simulink model "Bixler"  (R2019b)
settings: Solver=ode45  StartTime=0.0  StopTime=60  RelTol=1e-6  AbsTol=1e-8
PostLoadFcn:
  | parameters_main
  | write_init_cond
StartFcn:
  | write_init_cond
  | disp('Simulating...');
StopFcn:
  | timetime = datestr(datetime('now','Format','hh:mm'));
  | disp(['End of Simulation.       ', timetime]);
  | clear timetime
undefined symbols (not defined in the file): Aero, APlane, Bxl, C, Ctr, deg, DiscIntNeverNeededParam, Earth, F, Guid, Init, Light, MIL, Path, rad, s, Trim, Utility, WGS84
libraries: aerolibconvert2 x39, simulink x14, dspsigops x6, simulink_extras x3, aerolibtransform2 x2, aerolibasang x2, aerolibfltsims x2, shared6dof x1, aerolibadyn x1, aerolibwind2 x1, aerolibanim x1, realtime_pacer_lib x1
(part 4 of 5)

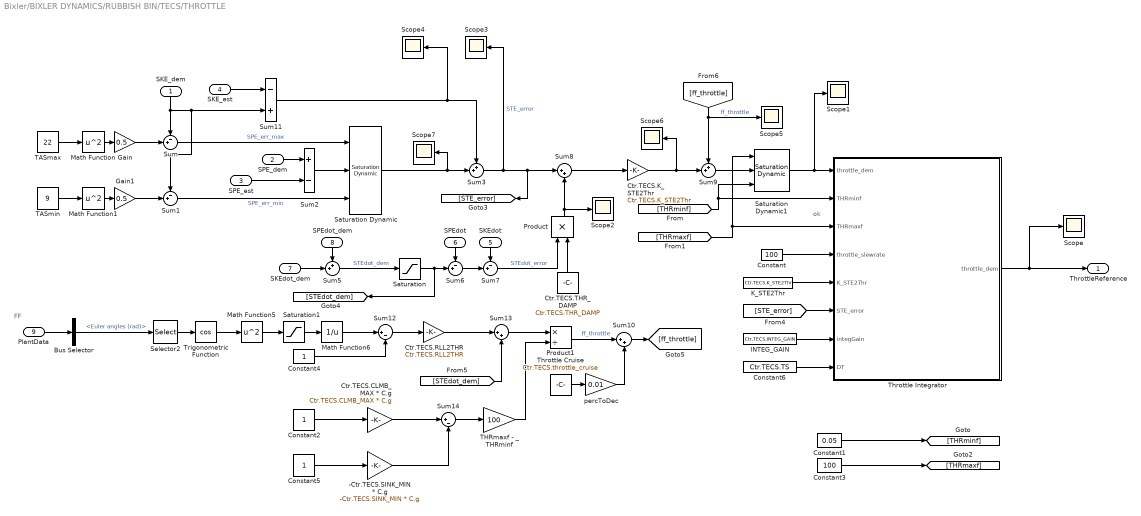
== system Bixler/BIXLER DYNAMICS/RUBBISH BIN/TECS/THROTTLE ==
  note: FF
  note: ok
  SKE_dem : Inport
  SPE_dem : Inport  Port=2
  SPE_est : Inport  Port=3
  SKE_est : Inport  Port=4
  SKEdot : Inport  Port=5
  SPEdot : Inport  Port=6
  SKEdot_dem : Inport  Port=7
  SPEdot_dem : Inport  Port=8
  PlantData : Inport  Port=9
  -Ctr.TECS.SINK_MIN * C.g : Gain  Gain=-Ctr.TECS.SINK_MIN * C.g
  Bus Selector : BusSelector  OutputSignals=Euler angles (rad)
  Constant : Constant  Value=100
  Constant1 : Constant  Value=0.05
  Constant2 : Constant
  Constant3 : Constant  Value=100
  Constant4 : Constant
  Constant5 : Constant
  Constant6 : Constant  Value=Ctr.TECS.TS
  Ctr.TECS.CLMB_MAX * C.g : Gain  Gain=Ctr.TECS.CLMB_MAX * C.g
  Ctr.TECS.K_STE2Thr : Gain  Gain=Ctr.TECS.K_STE2Thr
  Ctr.TECS.RLL2THR : Gain  Gain=Ctr.TECS.RLL2THR
  Ctr.TECS.THR_DAMP : Constant  Value=Ctr.TECS.THR_DAMP
  Gain : Gain  Gain=0.5
  Gain1 : Gain  Gain=0.5
  INTEG_GAIN : Constant  Value=Ctr.TECS.INTEG_GAIN
  K_STE2Thr : Constant  Value=Ctr.TECS.K_STE2Thr
  Math Function : Math  Operator=square  SignedPower=on  SaturateOnIntegerOverflow=on
  Math Function1 : Math  Operator=square  SignedPower=on  SaturateOnIntegerOverflow=on
  Math Function5 : Math  Operator=square  SignedPower=on  SaturateOnIntegerOverflow=on
  Math Function6 : Math  Operator=reciprocal  SignedPower=on  SaturateOnIntegerOverflow=on
  Product : Product
  Product1 : Product  Inputs=*/
  Saturation : Saturate  UpperLimit=Ctr.TECS.STEdot_max  LowerLimit=Ctr.TECS.STEdot_min
  Saturation Dynamic : simulink/Discontinuities/Saturation Dynamic  OutMin=[]  OutMax=[]  OutDataTypeStr=Inherit: Same as second input  OutDataType=fixdt(1, 16)  OutScaling=2^-10  DoSatur=off
  Saturation Dynamic1 : simulink/Discontinuities/Saturation Dynamic  OutMin=[]  OutMax=[]  OutDataTypeStr=Inherit: Same as second input  OutDataType=fixdt(1, 16)  OutScaling=2^-10  DoSatur=off
  Saturation1 : Saturate  UpperLimit=1  LowerLimit=0.1
  Scope{,1..7} (8 alike) : Scope
  Selector2 : Selector  InputPortWidth=3  IndexOptions=Index vector (dialog)  Indices=1  OutputSizes=1
  Sum{,1,6..7} (4 alike) : Sum  Inputs=-+|
  Sum10 : Sum  Inputs=|++
  Sum11 : Sum  Inputs=-+
  Sum12 : Sum  Inputs=|+-
  Sum13 : Sum  Inputs=|++
  Sum14 : Sum  Inputs=|+-
  Sum2 : Sum  Inputs=+-
  Sum3 : Sum  Inputs=++|
  Sum5 : Sum  Inputs=++|
  Sum8 : Sum  Inputs=|++
  Sum9 : Sum  Inputs=++|
  TASmax : Constant  Value=22
  TASmin : Constant  Value=9
  THRmaxf - _THRminf : Gain  Gain=100
  Throttle Cruise : Constant  Value=Ctr.TECS.throttle_cruise
  Throttle Integrator : MATLAB Function  TreatAsAtomicUnit=on
  Trigonometric Function : Trigonometry  Operator=cos
  percToDec : Gain  Gain=0.01
  ThrottleReference : Outport  VectorParamsAs1DForOutWhenUnconnected=off
  wires:
  Throttle Integrator/1(throttle_dem) -> Scope/1, ThrottleReference/1
  Constant6/1 -> Throttle Integrator/8(DT)
  SKE_dem/1 -> Sum11/2, Sum1/1, Sum/1
  Math Function1/1 -> Gain1/1
  TASmin/1 -> Math Function1/1
  Sum1/1 -> Saturation Dynamic/3  "SPE_err_min"
  Gain1/1 -> Sum1/2
  TASmax/1 -> Math Function/1
  Sum5/1 -> Saturation/1  "STEdot_dem"
  SPEdot/1 -> Sum6/1
  Saturation Dynamic1/1 -> Scope1/1, Throttle Integrator/1("throttle_dem ")
  Product/1 -> Sum8/2, Scope2/1
  Saturation/1 -> [STEdot_dem], Sum6/2
  Ctr.TECS.THR_DAMP/1 -> Product/2
  SPE_est/1 -> Sum2/2
  Sum6/1 -> Sum7/2
  Sum3/1 -> Scope3/1, [STE_error], Sum8/1  "STE_error"
  SPEdot_dem/1 -> Sum5/1
  SKEdot_dem/1 -> Sum5/2
  SKE_est/1 -> Sum11/1
  Sum7/1 -> Product/1  "STEdot_error"
  Sum2/1 -> Saturation Dynamic/2
  SKEdot/1 -> Sum7/1
  Sum9/1 -> Saturation Dynamic1/2
  Sum/1 -> Saturation Dynamic/1  "SPE_err_max"
  Gain/1 -> Sum/2
  Math Function/1 -> Gain/1
  Constant1/1 -> [THRminf]
  Constant3/1 -> [THRmaxf]
  [THRminf] -> Throttle Integrator/2(THRminf), Saturation Dynamic1/3
  [THRmaxf] -> Saturation Dynamic1/1, Throttle Integrator/3(THRmaxf)
  Constant/1 -> Throttle Integrator/4(throttle_slewrate)
  [STE_error] -> Throttle Integrator/6(STE_error)
  INTEG_GAIN/1 -> Throttle Integrator/7(integGain)
  SPE_dem/1 -> Sum2/1
  PlantData/1 -> Bus Selector/1
  Bus Selector/1 -> Selector2/1  "<Euler angles (rad)>"
  Selector2/1 -> Trigonometric Function/1
  Saturation1/1 -> Math Function6/1
  Math Function6/1 -> Sum12/1
  Constant4/1 -> Sum12/2
  Sum12/1 -> Ctr.TECS.RLL2THR/1
  Ctr.TECS.RLL2THR/1 -> Sum13/1
  [STEdot_dem] -> Sum13/2
  Ctr.TECS.K_STE2Thr/1 -> Scope6/1, Sum9/2
  K_STE2Thr/1 -> Throttle Integrator/5(K_STE2Thr)
  [ff_throttle] -> Sum9/1, Scope5/1  "ff_throttle"
  Sum8/1 -> Ctr.TECS.K_STE2Thr/1
  Math Function5/1 -> Saturation1/1
  Sum13/1 -> Product1/1
  Throttle Cruise/1 -> percToDec/1
  Constant2/1 -> Ctr.TECS.CLMB_MAX * C.g/1
  Constant5/1 -> -Ctr.TECS.SINK_MIN * C.g/1
  Ctr.TECS.CLMB_MAX * C.g/1 -> Sum14/1
  -Ctr.TECS.SINK_MIN * C.g/1 -> Sum14/2
  Sum14/1 -> THRmaxf - _THRminf/1
  THRmaxf - _THRminf/1 -> Product1/2
  Product1/1 -> Sum10/1  "ff_throttle"
  Sum10/1 -> [ff_throttle]
  Sum11/1 -> Scope4/1, Sum3/1
  Saturation Dynamic/1 -> Scope7/1, Sum3/2
  percToDec/1 -> Sum10/2
  Trigonometric Function/1 -> Math Function5/1

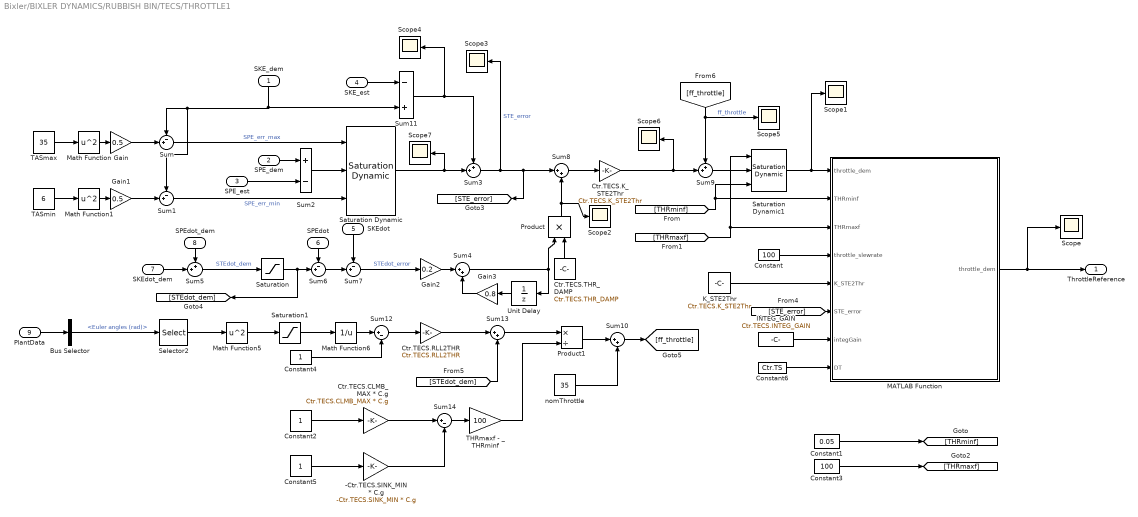
== system Bixler/BIXLER DYNAMICS/RUBBISH BIN/TECS/THROTTLE1 ==
  SKE_dem : Inport
  SPE_dem : Inport  Port=2
  SPE_est : Inport  Port=3
  SKE_est : Inport  Port=4
  SKEdot : Inport  Port=5
  SPEdot : Inport  Port=6
  SKEdot_dem : Inport  Port=7
  SPEdot_dem : Inport  Port=8
  PlantData : Inport  Port=9
  -Ctr.TECS.SINK_MIN * C.g : Gain  Gain=-Ctr.TECS.SINK_MIN * C.g
  Bus Selector : BusSelector  OutputSignals=Euler angles (rad)
  Constant : Constant  Value=100
  Constant1 : Constant  Value=0.05
  Constant2 : Constant
  Constant3 : Constant  Value=100
  Constant4 : Constant
  Constant5 : Constant
  Constant6 : Constant  Value=Ctr.TS
  Ctr.TECS.CLMB_MAX * C.g : Gain  Gain=Ctr.TECS.CLMB_MAX * C.g
  Ctr.TECS.K_STE2Thr : Gain  Gain=Ctr.TECS.K_STE2Thr
  Ctr.TECS.RLL2THR : Gain  Gain=Ctr.TECS.RLL2THR
  Ctr.TECS.THR_DAMP : Constant  Value=Ctr.TECS.THR_DAMP
  Gain : Gain  Gain=0.5
  Gain1 : Gain  Gain=0.5
  Gain2 : Gain  Gain=0.2
  Gain3 : Gain  Gain=0.8
  INTEG_GAIN : Constant  Value=Ctr.TECS.INTEG_GAIN
  K_STE2Thr : Constant  Value=Ctr.TECS.K_STE2Thr
  MATLAB Function : MATLAB Function  TreatAsAtomicUnit=on
  Math Function : Math  Operator=square  SignedPower=on  SaturateOnIntegerOverflow=on
  Math Function1 : Math  Operator=square  SignedPower=on  SaturateOnIntegerOverflow=on
  Math Function5 : Math  Operator=square  SignedPower=on  SaturateOnIntegerOverflow=on
  Math Function6 : Math  Operator=reciprocal  SignedPower=on  SaturateOnIntegerOverflow=on
  Product : Product
  Product1 : Product  Inputs=*/
  Saturation : Saturate  UpperLimit=Ctr.TECS.STEdot_max  LowerLimit=Ctr.TECS.STEdot_min
  Saturation Dynamic : simulink/Discontinuities/Saturation Dynamic  OutMin=[]  OutMax=[]  OutDataTypeStr=Inherit: Same as second input  OutDataType=fixdt(1, 16)  OutScaling=2^-10  DoSatur=off
  Saturation Dynamic1 : simulink/Discontinuities/Saturation Dynamic  OutMin=[]  OutMax=[]  OutDataTypeStr=Inherit: Same as second input  OutDataType=fixdt(1, 16)  OutScaling=2^-10  DoSatur=off
  Saturation1 : Saturate  UpperLimit=1  LowerLimit=0.1
  Scope{,1..7} (8 alike) : Scope
  Selector2 : Selector  InputPortWidth=3  IndexOptions=Index vector (dialog)  Indices=1  OutputSizes=1
  Sum{,1,6..7} (4 alike) : Sum  Inputs=-+|
  Sum{4,8,10,13} (4 alike) : Sum  Inputs=|++
  Sum11 : Sum  Inputs=-+
  Sum12 : Sum  Inputs=|+-
  Sum14 : Sum  Inputs=|+-
  Sum2 : Sum  Inputs=+-
  Sum3 : Sum  Inputs=++|
  Sum5 : Sum  Inputs=++|
  Sum9 : Sum  Inputs=++|
  TASmax : Constant  Value=35
  TASmin : Constant  Value=6
  THRmaxf - _THRminf : Gain  Gain=100
  Unit Delay : UnitDelay  SampleTime=Ctr.TS  HasFrameUpgradeWarning=on
  nomThrottle : Constant  Value=35
  ThrottleReference : Outport  VectorParamsAs1DForOutWhenUnconnected=off
  wires:
  MATLAB Function/1(throttle_dem) -> Scope/1, ThrottleReference/1
  Constant6/1 -> MATLAB Function/8(DT)
  SKE_dem/1 -> Sum/1, Sum1/1, Sum11/2
  Math Function1/1 -> Gain1/1
  TASmin/1 -> Math Function1/1
  Sum1/1 -> Saturation Dynamic/3  "SPE_err_min"
  Gain1/1 -> Sum1/2
  TASmax/1 -> Math Function/1
  Sum5/1 -> Saturation/1  "STEdot_dem"
  SPEdot/1 -> Sum6/1
  Saturation Dynamic1/1 -> Scope1/1, MATLAB Function/1("throttle_dem ")
  Product/1 -> Scope2/1, Sum8/2
  Saturation/1 -> [STEdot_dem], Sum6/2
  Ctr.TECS.THR_DAMP/1 -> Product/2
  SPE_est/1 -> Sum2/2
  Sum6/1 -> Sum7/2
  Sum3/1 -> Scope3/1, [STE_error], Sum8/1  "STE_error"
  SPEdot_dem/1 -> Sum5/1
  SKEdot_dem/1 -> Sum5/2
  SKE_est/1 -> Sum11/1
  Sum7/1 -> Gain2/1  "STEdot_error"
  Sum2/1 -> Saturation Dynamic/2
  SKEdot/1 -> Sum7/1
  Sum9/1 -> Saturation Dynamic1/2
  Sum/1 -> Saturation Dynamic/1  "SPE_err_max"
  Gain/1 -> Sum/2
  Math Function/1 -> Gain/1
  Constant1/1 -> [THRminf]
  Constant3/1 -> [THRmaxf]
  [THRminf] -> MATLAB Function/2(THRminf), Saturation Dynamic1/3
  [THRmaxf] -> Saturation Dynamic1/1, MATLAB Function/3(THRmaxf)
  Constant/1 -> MATLAB Function/4(throttle_slewrate)
  [STE_error] -> MATLAB Function/6(STE_error)
  INTEG_GAIN/1 -> MATLAB Function/7(integGain)
  SPE_dem/1 -> Sum2/1
  PlantData/1 -> Bus Selector/1
  Bus Selector/1 -> Selector2/1  "<Euler angles (rad)>"
  Selector2/1 -> Math Function5/1
  Saturation1/1 -> Math Function6/1
  Math Function6/1 -> Sum12/1
  Constant4/1 -> Sum12/2
  Sum12/1 -> Ctr.TECS.RLL2THR/1
  Ctr.TECS.RLL2THR/1 -> Sum13/1
  [STEdot_dem] -> Sum13/2
  Ctr.TECS.K_STE2Thr/1 -> Scope6/1, Sum9/2
  K_STE2Thr/1 -> MATLAB Function/5(K_STE2Thr)
  [ff_throttle] -> Sum9/1, Scope5/1  "ff_throttle"
  Sum8/1 -> Ctr.TECS.K_STE2Thr/1
  Math Function5/1 -> Saturation1/1
  Sum13/1 -> Product1/1
  nomThrottle/1 -> Sum10/2
  Constant2/1 -> Ctr.TECS.CLMB_MAX * C.g/1
  Constant5/1 -> -Ctr.TECS.SINK_MIN * C.g/1
  Ctr.TECS.CLMB_MAX * C.g/1 -> Sum14/1
  -Ctr.TECS.SINK_MIN * C.g/1 -> Sum14/2
  Sum14/1 -> THRmaxf - _THRminf/1
  THRmaxf - _THRminf/1 -> Product1/2
  Product1/1 -> Sum10/1
  Sum10/1 -> [ff_throttle]
  Sum11/1 -> Scope4/1, Sum3/1
  Gain2/1 -> Sum4/1
  Gain3/1 -> Sum4/2
  Unit Delay/1 -> Gain3/1
  Sum4/1 -> Unit Delay/1, Product/1
  Saturation Dynamic/1 -> Scope7/1, Sum3/2

== system Bixler/BIXLER DYNAMICS/Vehicle Airframe/Aerodynamics/Aerodynamic Coefficients ==
  PlantData : Inport
  Va : Inport  Port=2
  alpha(rad) : Inport  Port=3
  beta(rad) : Inport  Port=4
  Alpha Prelookup : PreLookup  BreakpointsData=Aero.alpha_vector  BeginIndexSearchUsingPreviousIndexResult=on  ExtrapMethod=Linear  RemoveProtectionInput=on
  Angle Conversion : aerolibconvert2/Angle Conversion  IU=rad  OU=deg
  Bus Selector : BusSelector  OutputSignals=Angular rates (body) (rad/s)
  Demux1 : Demux  Outputs=3
  Forces : Subsystem
  Goto Tag Visibility : GotoTagVisibility  GotoTag=pRad
  Goto Tag Visibility1 : GotoTagVisibility  GotoTag=qRad
  Goto Tag Visibility2 : GotoTagVisibility  GotoTag=rRad
  Goto Tag Visibility3 : GotoTagVisibility  GotoTag=BetaRad
  Moments : Subsystem
  Mux : Mux  Inputs=6
  Coeff : Outport  VectorParamsAs1DForOutWhenUnconnected=off
  tag scope: BetaRad=scoped, Va=global, alphaRad=scoped, pRad=scoped, qRad=scoped, rRad=scoped
  wires:
  Alpha Prelookup/2 -> Moments/2(alpha_f), Forces/2(alpha_f)  "f"
  alpha(rad)/1 -> [alphaRad], Angle Conversion/1
  PlantData/1 -> Bus Selector/1
  Forces/1(CD) -> Mux/1
  Forces/2(Cy) -> Mux/2
  Moments/1(Cl) -> Mux/4
  Demux1/3 -> [rRad]  "yaw_rate"
  Angle Conversion/1 -> Alpha Prelookup/1
  Demux1/2 -> [qRad]  "pitch_rate"
  beta(rad)/1 -> [BetaRad]
  Alpha Prelookup/1 -> Moments/1(alpha_k), Forces/1(alpha_k)  "k"
  Demux1/1 -> [pRad]  "roll_rate"
  Forces/3(CL) -> Mux/3
  Moments/3(Cn) -> Mux/6
  Moments/2(Cm) -> Mux/5
  Mux/1 -> Coeff/1
  Bus Selector/1 -> Demux1/1  "<Angular rates (body) (rad/s)>"
  Va/1 -> [Va]

== system Bixler/BIXLER DYNAMICS/Vehicle Airframe/Aerodynamics/ControlIncrements ==
  DerCond : Inport
  Control : Inport  Port=2
  Ailerons : Subsystem
  Alpha : PreLookup  BreakpointsData=Aero.alpha_vector  BeginIndexSearchUsingPreviousIndexResult=on  ExtrapMethod=Linear  RemoveProtectionInput=on
  Angle Conversion : aerolibconvert2/Angle Conversion  IU=rad  OU=deg
  Bus Selector : BusSelector  OutputSignals=alpha
  Bus Selector1 : BusSelector  OutputSignals=delta_ail,delta_elev,delta_rudd
  Elevator : Subsystem
  Rudder : Subsystem
  Cn_ail : Outport  VectorParamsAs1DForOutWhenUnconnected=off
  Cl_ail : Outport  Port=2  VectorParamsAs1DForOutWhenUnconnected=off
  CD_elev : Outport  Port=3  VectorParamsAs1DForOutWhenUnconnected=off
  CL_elev : Outport  Port=4  VectorParamsAs1DForOutWhenUnconnected=off
  Cm_elev : Outport  Port=5  VectorParamsAs1DForOutWhenUnconnected=off
  Cy_rudd : Outport  Port=6  VectorParamsAs1DForOutWhenUnconnected=off
  Cl_rudd : Outport  Port=7  VectorParamsAs1DForOutWhenUnconnected=off
  Cn_rudd : Outport  Port=8  VectorParamsAs1DForOutWhenUnconnected=off
  wires:
  Rudder/3(Cn_rudd) -> Cn_rudd/1
  Rudder/2(Cl_rudd) -> Cl_rudd/1
  Rudder/1(Cy_rudd) -> Cy_rudd/1
  Elevator/3(Cm_elev) -> Cm_elev/1
  Elevator/2(CL_elev) -> CL_elev/1
  Elevator/1(CD_elev) -> CD_elev/1
  Angle Conversion/1 -> Alpha/1
  Ailerons/2(Cl_ail) -> Cl_ail/1
  Ailerons/1(Cn_ail) -> Cn_ail/1
  Bus Selector1/3 -> Rudder/1(deltaRudd)  "<delta_rudd>"
  Bus Selector1/2 -> Elevator/3(DeltaElev)  "<delta_elev>"
  Alpha/2 -> Ailerons/2(alpha_f), Elevator/2(alpha_f)
  Alpha/1 -> Ailerons/1(alpha_k), Elevator/1(alpha_k)
  Bus Selector1/1 -> Ailerons/3(DeltaAil)  "<delta_ail>"
  Bus Selector/1 -> Angle Conversion/1  "<alpha>"
  DerCond/1 -> Bus Selector/1
  Control/1 -> Bus Selector1/1

== system Bixler/BIXLER DYNAMICS/Vehicle Airframe/Aerodynamics/Forces//Moments ==
  note: From stability frame to body frame
  CD : Inport
  Cy : Inport  Port=2
  CL : Inport  Port=3
  Cl : Inport  Port=4
  Cm : Inport  Port=5
  Cn : Inport  Port=6
  DerCond : Inport  Port=7
  "Aerodynamic Forces and Moments " : aerolibadyn/Aerodynamic Forces and Moments   inputAxes=Body  outputForceAxes=Body  outputMomentAxes=Body  S=Bxl.S  b=Bxl.c  cbar=Bxl.b
  Bus Selector : BusSelector  OutputSignals=qbar
  Constant : Constant  Value=Bxl.COG
  Demux : Demux  Outputs=3
  From wind to body : Math  Operator=transpose  SignedPower=on  SaturateOnIntegerOverflow=on
  Gain2 : Gain  Gain=-1
  Gain3 : Gain  Gain=-1
  Manual Switch : ManualSwitch  CurrentSetting=0
  Mux : Mux  Inputs=6
  Mux1 : Mux  Inputs=3
  Mux3 : Mux  Inputs=2
  Product : Product  Inputs=**  Multiplication=Matrix(*)
  Rotation Matrix Body to Wind : aerolibtransform2/Direction Cosine Matrix Body to Wind
      settings: SourceProductBaseCode=AE
  beta : Constant  Value=0
  neglect center of gravity and center of pressure effects : Constant  Value=[0 0 0]
  Fxyz : Outport  VectorParamsAs1DForOutWhenUnconnected=off
  Mlmn : Outport  Port=2  VectorParamsAs1DForOutWhenUnconnected=off
  wires:
  Demux/1 -> Mux/1  "Cx"
  Demux/3 -> Mux/3  "Cz"
  Mux/1 -> "Aerodynamic Forces and Moments "/1
  Cn/1 -> Mux/6
  CD/1 -> Gain2/1
  Cl/1 -> Mux/4
  Mux1/1 -> Product/2
  Constant/1 -> Manual Switch/1
  "Aerodynamic Forces and Moments "/2 -> Mlmn/1
  "Aerodynamic Forces and Moments "/1 -> Fxyz/1
  Bus Selector/1 -> "Aerodynamic Forces and Moments "/2  "<qbar>"
  DerCond/1 -> Bus Selector/1
  CL/1 -> Gain3/1
  Cm/1 -> Mux/5
  [alphaRad] -> Mux3/1
  beta/1 -> Mux3/2
  Mux3/1 -> Rotation Matrix Body to Wind/1
  Rotation Matrix Body to Wind/1 -> From wind to body/1
  Gain2/1 -> Mux1/1
  Gain3/1 -> Mux1/3
  Cy/1 -> Mux1/2
  From wind to body/1 -> Product/1
  Product/1 -> Demux/1
  Demux/2 -> Mux/2  "Cy"
  neglect center of gravity and center of pressure effects/1 -> Manual Switch/2
  Manual Switch/1 -> "Aerodynamic Forces and Moments "/4, "Aerodynamic Forces and Moments "/3

== system Bixler/BIXLER DYNAMICS/Vehicle Airframe/Propulsion/By interpolation ==
  In1 : Inport
  Prelookup : PreLookup  BreakpointsData=Aero.thrust_vect  BeginIndexSearchUsingPreviousIndexResult=on  RemoveProtectionInput=on
  Throttle interpolation : Interpolation_n-D  NumberOfTableDimensions=1  Table=Aero.thrust_force_vect  ExtrapMethod=Clip  RemoveProtectionIndex=on  InternalRulePriority=Speed
      settings: InputPortMap=u0,u1
  Out1 : Outport  VectorParamsAs1DForOutWhenUnconnected=off
  wires:
  Prelookup/1 -> Throttle interpolation/1
  Prelookup/2 -> Throttle interpolation/2
  Throttle interpolation/1 -> Out1/1
  In1/1 -> Prelookup/1

== system Bixler/BIXLER DYNAMICS/Vehicle Airframe/Propulsion/Propeller model (Bernoulli) ==
  DerCond : Inport
  Throttle : Inport  Port=2
  0.5 * C.rho * Bxl.S_prop * Bxl.rotor_thrust_coeff : Gain  Gain=0.5 * C.rho * Bxl.S_prop * Bxl.rotor_thrust_coeff
  Bus Selector : BusSelector  OutputSignals=Va
  Bxl.r_prop : Gain  Gain=Bxl.r_prop*0.5
  Math Function : Math  Operator=square  SignedPower=on  SaturateOnIntegerOverflow=on
  Math Function1 : Math  Operator=square  SignedPower=on  SaturateOnIntegerOverflow=on
  Sum : Sum  Inputs=+-
  k_motor * u + q_motor : Fcn  Expr=Bxl.k_motor * u + Bxl.q_motor
  Thrust : Outport  VectorParamsAs1DForOutWhenUnconnected=off
  wires:
  Math Function/1 -> Sum/2  "V_a^2"
  Sum/1 -> 0.5 * C.rho * Bxl.S_prop * Bxl.rotor_thrust_coeff/1
  DerCond/1 -> Bus Selector/1
  Throttle/1 -> k_motor * u + q_motor/1
  0.5 * C.rho * Bxl.S_prop * Bxl.rotor_thrust_coeff/1 -> Thrust/1  "T"
  Bxl.r_prop/1 -> Math Function1/1  "Air flow velocity after prop."
  k_motor * u + q_motor/1 -> Bxl.r_prop/1  "Prop. angular speed (Omega)"
  Math Function1/1 -> Sum/1  "(R*Ome)^2"
  Bus Selector/1 -> Math Function/1  "<Va>"

== system Bixler/PATH FOLLOWING/Orbit Path Following (Enabled Subsystem)/Loiter Controller/Parameters Mixer ==
  Constant1 : Constant  Value=Guid.Est.alpha
  Constant6 : Constant  Value=Guid.Loiter.k
  Constant7 : Constant  Value=Guid.Loiter.kk
  Constant8 : Constant  Value=Guid.Loiter.eps
  Mux : Mux  Inputs=6
  param : Outport  VectorParamsAs1DForOutWhenUnconnected=off
  wires:
  Mux/1 -> param/1
  Constant6/1 -> Mux/1
  Constant7/1 -> Mux/2
  Constant8/1 -> Mux/3
  [R] -> Mux/4
  [j] -> Mux/5
  Constant1/1 -> Mux/6

== system Bixler/PATH FOLLOWING/Orbit Path Following (Enabled Subsystem)/Vg Estimator/Parameters Mixer1 ==
  airspeed : Inport
  Constant : Constant  Value=Guid.Wind.W
  Constant1 : Constant  Value=Guid.Wind.phiw
  Constant11 : Constant  Value=Guid.Loiter.gamma
  Constant2 : Constant  Value=Guid.Loiter.d_int
  Constant3 : Constant  Value=Guid.Loiter.sigma
  Constant6 : Constant  Value=Guid.Loiter.k
  Constant7 : Constant  Value=Guid.Loiter.kk
  Constant8 : Constant  Value=Guid.Loiter.eps
  From27 : From  Commented=on  GotoTag=Target_Airspeed  TagVisibility=global
  Mux : Mux  Inputs=11
  param : Outport  VectorParamsAs1DForOutWhenUnconnected=off
  wires:
  Constant11/1 -> Mux/10
  [R] -> Mux/8
  Mux/1 -> param/1
  [j] -> Mux/9
  Constant/1 -> Mux/1
  Constant8/1 -> Mux/6
  Constant6/1 -> Mux/4
  Constant7/1 -> Mux/5
  airspeed/1 -> Mux/3
  Constant1/1 -> Mux/2
  Constant2/1 -> Mux/7
  Constant3/1 -> Mux/11

== system Bixler/PATH FOLLOWING/Straight-line Path Following (Enabled Subsystem)/SL.controller/Param. Mixer ==
  Constant1 : Constant  Value=Guid.SL.chi_inf
  Constant2 : Constant  Value=Guid.Est.alpha
  Constant3 : Constant  Value=Guid.SL.kk
  Constant4 : Constant  Value=Guid.SL.eps
  Constant5 : Constant  Value=Guid.SL.k
  Mux : Mux  Inputs=5
  param : Outport  VectorParamsAs1DForOutWhenUnconnected=off
  wires:
  Constant2/1 -> Mux/5  "alpha"
  Constant3/1 -> Mux/4  "kk"
  Constant5/1 -> Mux/3  "k"
  Constant1/1 -> Mux/2  "chi_inf"
  Constant4/1 -> Mux/1  "eps"
  Mux/1 -> param/1

== system Bixler/PATH FOLLOWING/Straight-line Path Following (Enabled Subsystem)/Vg Estimator/Param. Mixer ==
  Va : Inport
  Constant1 : Constant  Value=Guid.Wind.W
  Constant12 : Constant  Value=Guid.SL.gamma
  Constant2 : Constant  Value=Guid.Wind.phiw
  Constant3 : Constant  Value=Guid.SL.eps
  Constant4 : Constant  Value=Guid.SL.epy
  Constant5 : Constant  Value=Guid.SL.sigma
  Constant6 : Constant  Value=Guid.SL.chi_inf
  Constant7 : Constant  Value=Guid.SL.k
  Constant8 : Constant  Value=Guid.SL.kk
  Constant9 : Constant  Value=Guid.Est.alpha
  Mux : Mux  Inputs=11
  param : Outport  VectorParamsAs1DForOutWhenUnconnected=off
  wires:
  Mux/1 -> param/1
  Constant4/1 -> Mux/1  "y_int"
  Constant6/1 -> Mux/6  "chi_inf"
  Constant7/1 -> Mux/7  "k"
  Constant1/1 -> Mux/2  "W"
  Constant8/1 -> Mux/8  "kk"
  Constant3/1 -> Mux/4  "epsilon"
  Constant2/1 -> Mux/5  "phiw = constant wind direction"
  Constant12/1 -> Mux/9  "gamma"
  Constant5/1 -> Mux/10  "sigma"
  Va/1 -> Mux/3  "Va"
  Constant9/1 -> Mux/11  "alpha"

== system Bixler/AUTOPILOT/Low-level Controllers/Pitch controller/Coordination offset/cos ==
  In1 : Inport
  Trigonometric Function : Trigonometry  Operator=cos
  Out1 : Outport  VectorParamsAs1DForOutWhenUnconnected=off
  wires:
  In1/1 -> Trigonometric Function/1
  Trigonometric Function/1 -> Out1/1

== system Bixler/AUTOPILOT/Low-level Controllers/Pitch controller/Coordination offset/sin ==
  In1 : Inport
  Angle Conversion : aerolibconvert2/Angle Conversion  Commented=through  IU=deg  OU=rad
  Angle Conversion1 : aerolibconvert2/Angle Conversion  Commented=through  IU=rad  OU=deg
  Trigonometric Function : Trigonometry
  Out1 : Outport  VectorParamsAs1DForOutWhenUnconnected=off
  wires:
  Trigonometric Function/1 -> Angle Conversion1/1
  Angle Conversion/1 -> Trigonometric Function/1
  Angle Conversion1/1 -> Out1/1
  In1/1 -> Angle Conversion/1

== system Bixler/AUTOPILOT/Low-level Controllers/Pitch controller/Coordination offset/tan ==
  In1 : Inport
  Angle Conversion : aerolibconvert2/Angle Conversion  Commented=through  IU=deg  OU=rad
  Angle Conversion1 : aerolibconvert2/Angle Conversion  Commented=through  IU=rad  OU=deg
  Trigonometric Function : Trigonometry  Operator=tan
  Out1 : Outport  VectorParamsAs1DForOutWhenUnconnected=off
  wires:
  In1/1 -> Angle Conversion/1
  Angle Conversion1/1 -> Out1/1
  Angle Conversion/1 -> Trigonometric Function/1
  Trigonometric Function/1 -> Angle Conversion1/1

== system Bixler/AUTOPILOT/Low-level Controllers/Pitch controller/Pitch PID/Adjust integrator gain ==
  Constant10 : Constant  Value=0.15
  Ctr.Pitch.PTCH2SRV_TCONST : Gain  Gain=Ctr.Pitch.PTCH2SRV_TCONST
  MinMax : MinMax  Function=max  Inputs=2
  K_I rate : Outport  VectorParamsAs1DForOutWhenUnconnected=off
  wires:
  ? -> MinMax/1
  Ctr.Pitch.PTCH2SRV_TCONST/1 -> K_I rate/1  "ki_rate"
  Constant10/1 -> MinMax/2
  MinMax/1 -> Ctr.Pitch.PTCH2SRV_TCONST/1

== system Bixler/AUTOPILOT/Low-level Controllers/Pitch controller/Pitch PID/Anti-windup ==
  u : Inport
  y : Inport  Port=2
  If : If  IfExpression=u1 < -45  ElseIfExpressions=u1 > 45
  If Action Subsystem : Subsystem  TreatAsAtomicUnit=on
  If Action Subsystem1 : Subsystem  TreatAsAtomicUnit=on
  If Action Subsystem2 : Subsystem  TreatAsAtomicUnit=on
  Merge : Merge  Inputs=3
  y_int : Outport  VectorParamsAs1DForOutWhenUnconnected=off
  wires:
  If Action Subsystem1/1(Out1) -> Merge/2
  Merge/1 -> y_int/1
  If Action Subsystem2/1(Out1) -> Merge/3
  y/1 -> If/1
  If Action Subsystem/1(Out1) -> Merge/1
  u/1 -> If Action Subsystem/1(In1), If Action Subsystem1/1(In1), If Action Subsystem2/1(In1)
  If/2 -> If Action Subsystem1/Action
  If/1 -> If Action Subsystem/Action
  If/3 -> If Action Subsystem2/Action

== system Bixler/AUTOPILOT/Low-level Controllers/Pitch controller/Pitch PID/Subsystem ==
  In1 : Inport
  Meas_roll_angle : Inport  Port=2
  Meas_pitch_rate : Inport  Port=3  Unit=deg/s
  +-45 : Saturate  UpperLimit=45  LowerLimit=-45
  Abs : Abs
  Abs1 : Abs
  Gain : Gain  Gain=-1
  If : If  IfExpression=u1 > 90
  If Action Subsystem : Subsystem  TreatAsAtomicUnit=on
  If Action Subsystem1 : Subsystem  TreatAsAtomicUnit=on
  If Action Subsystem2 : Subsystem  TreatAsAtomicUnit=on
  If Action Subsystem3 : Subsystem  TreatAsAtomicUnit=on
  If1 : If  NumInputs=2  IfExpression=u1 >84 & u2 < 70
  Merge : Merge
  Merge1 : Merge
  Out1 : Outport  VectorParamsAs1DForOutWhenUnconnected=off
  wires:
  If Action Subsystem3/1(Out1) -> Merge1/2
  Abs/1 -> If Action Subsystem/1(In1), If Action Subsystem1/1(In1), If/1
  Meas_pitch_rate/1 -> Abs1/1
  If/1 -> If Action Subsystem/Action
  Merge/1 -> If Action Subsystem2/1(In1), If1/1  "roll wrapped"
  If Action Subsystem2/1(Out1) -> Merge1/1
  +-45/1 -> Gain/1
  If1/2 -> If Action Subsystem3/Action
  Abs1/1 -> If1/2
  If Action Subsystem1/1(Out1) -> Merge/2
  Meas_roll_angle/1 -> Abs/1
  If1/1 -> If Action Subsystem2/Action
  In1/1 -> If Action Subsystem3/1(In1), If Action Subsystem2/2(In2)
  Gain/1 -> Out1/1
  If Action Subsystem/1(Out1) -> Merge/1
  If/2 -> If Action Subsystem1/Action
  Merge1/1 -> [lastO], +-45/1

== system Bixler/AUTOPILOT/Low-level Controllers/Pitch controller/TRASH/If Action Subsystem ==
  Action Port : ActionPort  ActionPortLabel=if { }
  Constant : Constant  Value=0
  Out1 : Outport  VectorParamsAs1DForOutWhenUnconnected=off
  wires:
  Constant/1 -> Out1/1

== system Bixler/AUTOPILOT/Low-level Controllers/Pitch controller/TRASH/If Action Subsystem1 ==
  pitch : Inport
  bank : Inport  Port=2
  Va : Inport  Port=3
  Action Port : ActionPort  ActionPortLabel=else { }
  Abs : Abs
  Constant : Constant  Value=C.g
  Constant1 : Constant  Value=APlane.EAS2TAS
  Constant2 : Constant  Value=APlane.airspeed_min
  Constant3 : Constant  Value=Ctr.Pitch.PTCH2SRV_RLL
  MinMax : MinMax  Function=max  Inputs=2
  Product : Product  Inputs=***
  Product1 : Product  Inputs=*/**
  Product2 : Product  Inputs=**
  bank1 : InportShadow  Port=2
  cosd : Subsystem
  sind : Subsystem
  tand : Subsystem
  Out1 : Outport  VectorParamsAs1DForOutWhenUnconnected=off
  wires:
  Product/1 -> Out1/1
  Abs/1 -> Product/2
  Constant/1 -> Product1/1
  MinMax/1 -> Product1/2
  Constant1/1 -> Product2/2
  Va/1 -> Product2/1
  Product2/1 -> MinMax/1
  Constant2/1 -> MinMax/2
  cosd/1(Out1) -> Product/1
  bank/1 -> tand/1(In1)
  bank1/1 -> sind/1(In1)
  Product1/1 -> Abs/1
  pitch/1 -> cosd/1(In1)
  tand/1(Out1) -> Product1/3
  sind/1(Out1) -> Product1/4
  Constant3/1 -> Product/3

== system Bixler/AUTOPILOT/Low-level Controllers/Pitch controller/TRASH/Parameters mixer1 ==
  note: 9
  note: 8
  note: 7
  note: 6
  note: 5
  note: 4
  note: 3
  note: 2
  note: 1
  Constant : Constant  Value=Ctr.Pitch.PTCH2SRV_I
  Constant1 : Constant  Value=Ctr.Pitch.PTCH2SRV_D
  Constant2 : Constant  Value=Ctr.Pitch.PTCH2SRV_FF
  Constant3 : Constant  Value=Ctr.Pitch.PTCH2SRV_P
  Constant4 : Constant  Value=APlane.roll_limit
  Constant5 : Constant  Value=Ctr.Pitch.PTCH2SRV_IMAX
  Constant6 : Constant  Value=APlane.airspeed_min
  Constant7 : Constant  Value=APlane.EAS2TAS
  Constant8 : Constant  Value=Ctr.Pitch.PTCH2SRV_TCONST
  Mux : Mux  Inputs=9
  parameters : Outport  VectorParamsAs1DForOutWhenUnconnected=off
  wires:
  Mux/1 -> parameters/1
  Constant8/1 -> Mux/1
  Constant3/1 -> Mux/2
  Constant/1 -> Mux/3
  Constant1/1 -> Mux/4
  Constant5/1 -> Mux/5
  Constant2/1 -> Mux/6
  Constant6/1 -> Mux/7
  Constant7/1 -> Mux/8
  Constant4/1 -> Mux/9

== system Bixler/AUTOPILOT/Low-level Controllers/Pitch controller/TRASH/Parameters mixer2 ==
  Constant2 : Constant  Value=Ctr.Pitch.PTCH2SRV_RLL
  Constant3 : Constant  Value=C.g
  Constant5 : Constant  Value=APlane.EAS2TAS
  Constant6 : Constant  Value=APlane.airspeed_min
  Mux1 : Mux
  parameters_roll_comp : Outport  VectorParamsAs1DForOutWhenUnconnected=off
  wires:
  Constant6/1 -> Mux1/4
  Constant5/1 -> Mux1/3
  Mux1/1 -> parameters_roll_comp/1
  Constant3/1 -> Mux1/2
  Constant2/1 -> Mux1/1

== system Bixler/AUTOPILOT/Low-level Controllers/Roll controller/Roll Rate Controller/Anti-windup ==
  y : Inport
  u : Inport  Port=2
  If : If  IfExpression=u1 < -45  ElseIfExpressions=u1 > 45
  If Action Subsystem : Subsystem  TreatAsAtomicUnit=on
  If Action Subsystem1 : Subsystem  TreatAsAtomicUnit=on
  If Action Subsystem2 : Subsystem  TreatAsAtomicUnit=on
  Merge : Merge  Inputs=3
  y_int : Outport  VectorParamsAs1DForOutWhenUnconnected=off
  wires:
  If Action Subsystem1/1(Out1) -> Merge/2
  Merge/1 -> y_int/1
  If Action Subsystem2/1(Out1) -> Merge/3
  y/1 -> If/1
  If Action Subsystem/1(Out1) -> Merge/1
  u/1 -> If Action Subsystem/1(In1), If Action Subsystem1/1(In1), If Action Subsystem2/1(In1)
  If/2 -> If Action Subsystem1/Action
  If/1 -> If Action Subsystem/Action
  If/3 -> If Action Subsystem2/Action

== system Bixler/AUTOPILOT/Low-level Controllers/Roll controller/Roll Rate Controller/K_FF (real feedforward) ==
  Constant5 : Constant  Value=Ctr.Roll.RLL2SRV_FF
  Constant6 : Constant  Value=APlane.EAS2TAS
  Product1 : Product  Inputs=*/
  Out1 : Outport  VectorParamsAs1DForOutWhenUnconnected=off
  wires:
  Product1/1 -> Out1/1  "k_ff"
  Constant6/1 -> Product1/2
  Constant5/1 -> Product1/1

== system Bixler/AUTOPILOT/Low-level Controllers/Roll controller/Roll Rate Controller/K_P (feedforward) ==
  Constant : Constant  Value=APlane.EAS2TAS
  Constant2 : Constant  Value=0
  Constant7 : Constant  Value=Ctr.Roll.K_P
  MinMax : MinMax  Function=max  Inputs=2
  Product : Product  Inputs=*/
  Out1 : Outport  VectorParamsAs1DForOutWhenUnconnected=off
  wires:
  Constant2/1 -> MinMax/2
  Constant7/1 -> MinMax/1
  MinMax/1 -> Product/1
  Product/1 -> Out1/1  "kp_ff"
  Constant/1 -> Product/2

== system Bixler/BIXLER DYNAMICS/RUBBISH BIN/Straight Line/SL.controller/Param. Mixer ==
  Constant1 : Constant  Value=Guid.SL.chi_inf
  Constant2 : Constant  Value=Guid.Est.alpha
  Constant3 : Constant  Value=Guid.SL.kk
  Constant4 : Constant  Value=Guid.SL.eps
  Constant5 : Constant  Value=Guid.SL.k
  Mux : Mux  Inputs=5
  param : Outport  VectorParamsAs1DForOutWhenUnconnected=off
  wires:
  Constant2/1 -> Mux/5  "alpha"
  Constant3/1 -> Mux/4  "kk"
  Constant5/1 -> Mux/3  "k"
  Constant1/1 -> Mux/2  "chi_inf"
  Constant4/1 -> Mux/1  "eps"
  Mux/1 -> param/1

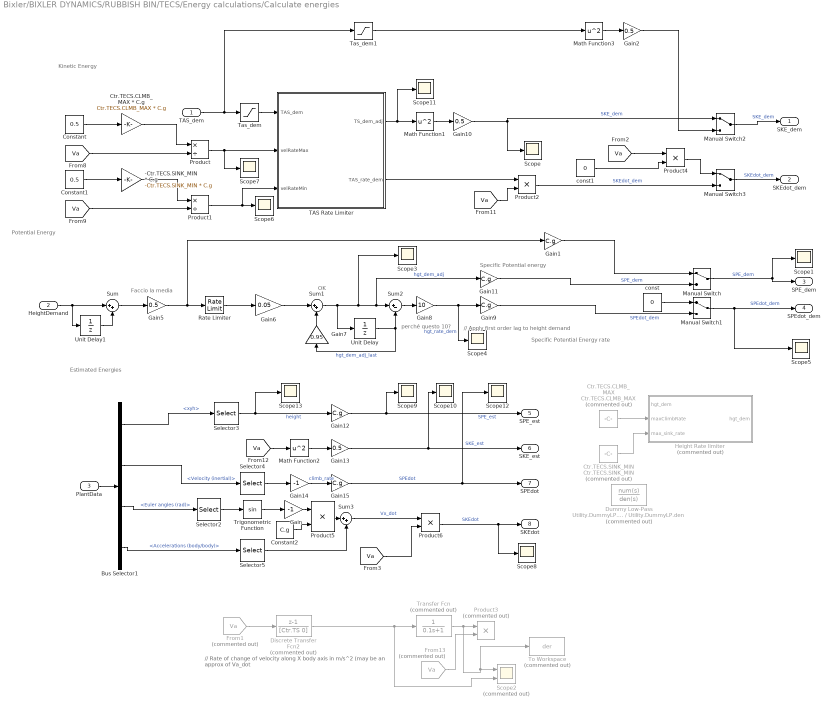
== system Bixler/BIXLER DYNAMICS/RUBBISH BIN/TECS/Energy calculations/Calculate energies ==
  note: Estimated Energies
  note: Potential Energy
  note: Kinetic Energy
  note: // Apply first order lag to height demand
  note: perché questo 10?
  note: Specific Potential Energy rate
  note: Specific Potential energy
  note: OK
  note: Faccio la media
  note: // Rate of change of velocity along X body axis in m/s^2
      | (may be an approx of Va_dot
  TAS_dem : Inport
  HeightDemand : Inport  Port=2
  PlantData : Inport  Port=3
  -Ctr.TECS.SINK_MIN * C.g : Gain  Gain=-Ctr.TECS.SINK_MIN * C.g
  Bus Selector1 : BusSelector  OutputSignals=xyh,Velocity (inertial),Euler angles (rad),Accelerations (body/body)
  Constant : Constant  Value=0.5
  Constant1 : Constant  Value=0.5
  Constant2 : Constant  Value=C.g
  Ctr.TECS.CLMB_MAX : Constant  Commented=on  Value=Ctr.TECS.CLMB_MAX
  Ctr.TECS.CLMB_MAX * C.g : Gain  Gain=Ctr.TECS.CLMB_MAX * C.g
  Ctr.TECS.SINK_MIN : Constant  Commented=on  Value=Ctr.TECS.SINK_MIN
  Discrete Transfer Fcn2 : DiscreteTransferFcn  Commented=on  Numerator=[1 -1]  Denominator=[Ctr.TS 0]  SampleTime=Ctr.TS
  Dummy Low-Pass : TransferFcn  Commented=on  Numerator=Utility.DummyLP.num  Denominator=Utility.DummyLP.den
  From1 : From  Commented=on  GotoTag=Va  TagVisibility=global
  From13 : From  Commented=on  GotoTag=Va  TagVisibility=global
  Gain : Gain  Gain=-1
  Gain{1,9,11..12,15} (5 alike) : Gain  Gain=C.g
  Gain{2,5,10,13} (4 alike) : Gain  Gain=0.5
  Gain14 : Gain  Gain=-1
  Gain6 : Gain  Gain=0.05
  Gain7 : Gain  Gain=0.95
  Gain8 : Gain  Gain=10
  Height Rate limiter : MATLAB Function  Commented=on  TreatAsAtomicUnit=on
  Manual Switch{,1..3} (4 alike) : ManualSwitch
  Math Function1 : Math  Operator=square  SignedPower=on  SaturateOnIntegerOverflow=on
  Math Function2 : Math  Operator=square  SignedPower=on  SaturateOnIntegerOverflow=on
  Math Function3 : Math  Operator=square  SignedPower=on  SaturateOnIntegerOverflow=on
  Product : Product  Inputs=*/
  Product1 : Product  Inputs=*/
  Product{2,4..6} (4 alike) : Product
  Product3 : Product  Commented=on
  Rate Limiter : RateLimiter  RisingSlewLimit=Ctr.TECS.CLMB_MAX  FallingSlewLimit=-Ctr.TECS.SINK_MIN  SampleTimeMode=inherited
  Scope{,1,3..13} (13 alike) : Scope
  Scope2 : Scope  Commented=on  NumInputPorts=2
  Selector2 : Selector  InputPortWidth=3  IndexOptions=Index vector (dialog)  Indices=2  OutputSizes=1
  Selector3 : Selector  InputPortWidth=3  IndexOptions=Index vector (dialog)  Indices=3  OutputSizes=1
  Selector4 : Selector  InputPortWidth=3  IndexOptions=Index vector (dialog)  Indices=3  OutputSizes=1
  Selector5 : Selector  InputPortWidth=3  IndexOptions=Index vector (dialog)  Indices=1  OutputSizes=1
  Sum : Sum  Inputs=|++
  Sum1 : Sum  Inputs=|++
  Sum2 : Sum  Inputs=|+-
  Sum3 : Sum  Inputs=|++
  TAS Rate Limiter : MATLAB Function  TreatAsAtomicUnit=on
  Tas_dem : Saturate  UpperLimit=35  LowerLimit=6
  Tas_dem1 : Saturate  UpperLimit=35  LowerLimit=6
  To Workspace : ToWorkspace  Commented=on  VariableName=der  SampleTime=-1
  Transfer Fcn : TransferFcn  Commented=on  Numerator=1  Denominator=[0.1 1]
  Trigonometric Function : Trigonometry
  Unit Delay : UnitDelay  SampleTime=Ctr.TS  HasFrameUpgradeWarning=on
  Unit Delay1 : UnitDelay  SampleTime=Ctr.TS  HasFrameUpgradeWarning=on
  const : Constant  Value=0
  const1 : Constant  Value=0
  SKE_dem : Outport  VectorParamsAs1DForOutWhenUnconnected=off
  SKEdot_dem : Outport  Port=2  VectorParamsAs1DForOutWhenUnconnected=off
  SPE_dem : Outport  Port=3  VectorParamsAs1DForOutWhenUnconnected=off
  SPEdot_dem : Outport  Port=4  VectorParamsAs1DForOutWhenUnconnected=off
  SPE_est : Outport  Port=5  VectorParamsAs1DForOutWhenUnconnected=off
  SKE_est : Outport  Port=6  VectorParamsAs1DForOutWhenUnconnected=off
  SPEdot : Outport  Port=7  VectorParamsAs1DForOutWhenUnconnected=off
  SKEdot : Outport  Port=8  VectorParamsAs1DForOutWhenUnconnected=off
  wires:
  Gain5/1 -> Gain1/1, Rate Limiter/1
  Gain8/1 -> Scope4/1, Gain9/1  "hgt_rate_dem"
  Gain6/1 -> Sum1/1
  Sum/1 -> Gain5/1
  Ctr.TECS.CLMB_MAX/1 -> Height Rate limiter/2(maxClimbRate)
  Ctr.TECS.SINK_MIN/1 -> Height Rate limiter/3(max_sink_rate)
  -Ctr.TECS.SINK_MIN * C.g/1 -> Product1/1
  Ctr.TECS.CLMB_MAX * C.g/1 -> Product/1
  Manual Switch/1 -> SPE_dem/1, Scope1/1  "SPE_dem"
  Sum2/1 -> Gain8/1
  Unit Delay/1 -> Gain7/1, Sum2/2  "hgt_dem_adj_last"
  Product2/1 -> Manual Switch3/2  "SKEdot_dem"
  Sum1/1 -> Unit Delay/1, Scope3/1, Gain11/1, Sum2/1  "hgt_dem_adj"
  Manual Switch1/1 -> Scope5/1, SPEdot_dem/1  "SPEdot_dem"
  [Va] -> Product2/2
  Gain12/1 -> Scope9/1, SPE_est/1  "SPE_est"
  Gain14/1 -> Gain15/1  "climb_rate"
  Gain13/1 -> Scope10/1, SKE_est/1  "SKE_est"
  TAS Rate Limiter/1(TS_dem_adj) -> Scope11/1, Math Function1/1
  Math Function2/1 -> Gain13/1
  TAS Rate Limiter/2(TAS_rate_dem) -> Product2/1
  Gain10/1 -> Manual Switch2/1, Scope/1  "SKE_dem"
  Math Function1/1 -> Gain10/1
  Selector3/1 -> Scope13/1, Gain12/1  "height"
  [Va] -> Math Function2/1
  Constant1/1 -> -Ctr.TECS.SINK_MIN * C.g/1
  Product1/1 -> Scope6/1, TAS Rate Limiter/3(velRateMin)
  Product/1 -> Scope7/1, TAS Rate Limiter/2(velRateMax)
  Gain7/1 -> Sum1/2
  Constant/1 -> Ctr.TECS.CLMB_MAX * C.g/1
  TAS_dem/1 -> Tas_dem1/1, Tas_dem/1
  HeightDemand/1 -> Unit Delay1/1, Sum/1
  Gain15/1 -> Scope12/1, SPEdot/1  "SPEdot"
  PlantData/1 -> Bus Selector1/1
  Bus Selector1/1 -> Selector3/1  "<xyh>"
  Bus Selector1/2 -> Selector4/1  "<Velocity (inertial)>"
  [Va] -> Product/2
  Selector4/1 -> Gain14/1
  [Va] -> Product1/2
  Rate Limiter/1 -> Gain6/1
  Unit Delay1/1 -> Sum/2
  Gain11/1 -> Manual Switch/2  "SPE_dem"
  Gain9/1 -> Manual Switch1/2  "SPEdot_dem"
  Gain1/1 -> Manual Switch/1
  Manual Switch2/1 -> SKE_dem/1  "SKE_dem"
  Math Function3/1 -> Gain2/1
  Gain2/1 -> Manual Switch2/2
  const1/1 -> Product4/2
  Tas_dem/1 -> TAS Rate Limiter/1(TAS_dem)
  [Va] -> Product4/1
  Product4/1 -> Manual Switch3/1
  Manual Switch3/1 -> SKEdot_dem/1  "SKEdot_dem"
  From13/1 -> Product3/2
  Product6/1 -> Scope8/1, SKEdot/1  "SKEdot"
  From1/1 -> Discrete Transfer Fcn2/1
  Discrete Transfer Fcn2/1 -> Transfer Fcn/1, Scope2/2
  Transfer Fcn/1 -> To Workspace/1, Scope2/1, Product3/1
  Bus Selector1/3 -> Selector2/1  "<Euler angles (rad)>"
  Sum3/1 -> Product6/1  "Vx_dot"
  [Va] -> Product6/2
  Selector2/1 -> Trigonometric Function/1
  Constant2/1 -> Product5/2
  Bus Selector1/4 -> Selector5/1  "<Accelerations (body/body)>"
  Product5/1 -> Sum3/1
  Selector5/1 -> Sum3/2
  Gain/1 -> Product5/1
  Trigonometric Function/1 -> Gain/1
  Tas_dem1/1 -> Math Function3/1
  const/1 -> Manual Switch1/1

== system Bixler/BIXLER DYNAMICS/RUBBISH BIN/TECS/PITCH/DT1 ==
  Clock1 : Clock
  Memory : Memory  InheritSampleTime=on
  Sum : Sum  Inputs=|+-
  DT : Outport  VectorParamsAs1DForOutWhenUnconnected=off
  wires:
  Memory/1 -> Sum/2
  Sum/1 -> DT/1
  Clock1/1 -> Memory/1, Sum/1

== system Bixler/BIXLER DYNAMICS/RUBBISH BIN/TECS/PITCH/Limiter ==
  integSEB_input : Inport
  PITCHmaxf : Inport  Port=2
  PITCHminf : Inport  Port=3
  pitch_dem : Inport  Port=4
  If : If  NumInputs=3  IfExpression=u1 > u2  ElseIfExpressions=u1 < u3
  If Action Subsystem : Subsystem  TreatAsAtomicUnit=on
  If Action Subsystem1 : Subsystem  TreatAsAtomicUnit=on
  If Action Subsystem2 : Subsystem  TreatAsAtomicUnit=on
  Merge : Merge  Inputs=3
  PITCHmaxf_1 : InportShadow  Port=2
  PITCHminf_1 : InportShadow  Port=3
  pitch_dem_1 : InportShadow  Port=4
  SEB_in_lim : Outport  VectorParamsAs1DForOutWhenUnconnected=off
  wires:
  If Action Subsystem1/1(Out1) -> Merge/3
  If Action Subsystem/1(Out1) -> Merge/1
  If Action Subsystem2/1(Out1) -> Merge/2
  PITCHminf_1/1 -> If Action Subsystem1/2(PITCHminf)
  integSEB_input/1 -> If/1, If Action Subsystem1/1(integSEB_input), If Action Subsystem2/1(integSEB_input), If Action Subsystem/1(integSEB_input)
  pitch_dem_1/1 -> If Action Subsystem1/3(pitch_dem)
  PITCHmaxf_1/1 -> If Action Subsystem/2(PITCHmaxf)
  If/3 -> If Action Subsystem2/Action
  PITCHmaxf/1 -> If/2
  Merge/1 -> SEB_in_lim/1
  PITCHminf/1 -> If/3
  pitch_dem/1 -> If Action Subsystem/3(pitch_dem)
  If/1 -> If Action Subsystem/Action
  If/2 -> If Action Subsystem1/Action

== system Bixler/BIXLER DYNAMICS/RUBBISH BIN/TECS/PITCH/integSEB ==
  temp : Inport
  gainInv : Inport  Port=2
  PITCHminf : Inport  Port=3
  PITCHmaxf : Inport  Port=4
  integSEB_delta : Inport  Port=5
  Constant : Constant  Value=0.0783
  Constant1 : Constant  Value=0.0783
  Gain : Gain  Gain=0.1
  Gain1 : Gain  Gain=-0.1
  Product : Product
  Product1 : Product
  Saturation Dynamic : simulink/Discontinuities/Saturation Dynamic  OutMin=[]  OutMax=[]  OutDataTypeStr=Inherit: Same as second input  OutDataType=fixdt(1, 16)  OutScaling=2^-10  DoSatur=off
  Sum : Sum  Inputs=|+-
  Sum1 : Sum  Inputs=|+-
  Sum2 : Sum  Inputs=|++
  Sum3 : Sum  Inputs=-+|
  Sum4 : Sum  Inputs=|+-
  gainInv_1 : InportShadow  Port=2
  "integSEB_min " : Outport  VectorParamsAs1DForOutWhenUnconnected=off
  "IntegSEB_delta " : Outport  Port=2  VectorParamsAs1DForOutWhenUnconnected=off
  integSEB_max : Outport  Port=3  VectorParamsAs1DForOutWhenUnconnected=off
  wires:
  PITCHminf/1 -> Sum/1
  Product/1 -> Sum1/1
  Constant1/1 -> Sum2/2
  Sum3/1 -> integSEB_max/1, [integSEB_max]
  PITCHmaxf/1 -> Sum2/1
  Sum2/1 -> Product1/2
  gainInv_1/1 -> Product1/1
  Constant/1 -> Sum/2
  integSEB_delta/1 -> Saturation Dynamic/2
  Sum/1 -> Product/2
  Sum1/1 -> "integSEB_min "/1, [integSEB_min]
  temp/1 -> Sum3/1, Sum1/2
  [integSEB_range] -> Gain1/1
  Gain1/1 -> Saturation Dynamic/3
  Saturation Dynamic/1 -> "IntegSEB_delta "/1
  Sum4/1 -> [integSEB_range]
  [integSEB_min] -> Sum4/2
  [integSEB_max] -> Sum4/1
  [integSEB_range] -> Gain/1
  Gain/1 -> Saturation Dynamic/1
  gainInv/1 -> Product/1
  Product1/1 -> Sum3/2

== system Bixler/BIXLER DYNAMICS/RUBBISH BIN/TECS/PITCH/timeConstant() ==
  Constant1 : Constant  Value=0.1
  Constant5 : Constant  Value=Ctr.TECS.TIME_CONST
  MinMax : MinMax  Function=max  Inputs=2
  timeConstant : Outport  VectorParamsAs1DForOutWhenUnconnected=off
  wires:
  MinMax/1 -> timeConstant/1
  Constant1/1 -> MinMax/2
  Constant5/1 -> MinMax/1

== system Bixler/BIXLER DYNAMICS/RUBBISH BIN/TECS/PITCH/timeConstant()1 ==
  Constant1 : Constant  Value=0.1
  Constant5 : Constant  Value=Ctr.TECS.TIME_CONST
  MinMax : MinMax  Function=max  Inputs=2
  timeConstant : Outport  VectorParamsAs1DForOutWhenUnconnected=off
  wires:
  MinMax/1 -> timeConstant/1
  Constant1/1 -> MinMax/2
  Constant5/1 -> MinMax/1

== system Bixler/BIXLER DYNAMICS/RUBBISH BIN/TECS/PITCH1/DT1 ==
  Clock1 : Clock
  Memory : Memory  InheritSampleTime=on
  Sum : Sum  Inputs=|+-
  DT : Outport  VectorParamsAs1DForOutWhenUnconnected=off
  wires:
  Memory/1 -> Sum/2
  Sum/1 -> DT/1
  Clock1/1 -> Memory/1, Sum/1

== system Bixler/BIXLER DYNAMICS/RUBBISH BIN/TECS/PITCH1/Limiter ==
  integSEB_input : Inport
  PITCHmaxf : Inport  Port=2
  PITCHminf : Inport  Port=3
  pitch_dem : Inport  Port=4
  If : If  NumInputs=3  IfExpression=u1 > u2  ElseIfExpressions=u1 < u3
  If Action Subsystem : Subsystem  TreatAsAtomicUnit=on
  If Action Subsystem1 : Subsystem  TreatAsAtomicUnit=on
  If Action Subsystem2 : Subsystem  TreatAsAtomicUnit=on
  Merge : Merge  Inputs=3
  PITCHmaxf_1 : InportShadow  Port=2
  PITCHminf_1 : InportShadow  Port=3
  pitch_dem_1 : InportShadow  Port=4
  y : Outport  VectorParamsAs1DForOutWhenUnconnected=off
  wires:
  If Action Subsystem1/1(Out1) -> Merge/3
  If Action Subsystem/1(Out1) -> Merge/1
  If Action Subsystem2/1(Out1) -> Merge/2
  PITCHminf_1/1 -> If Action Subsystem1/2(PITCHminf)
  integSEB_input/1 -> If/1, If Action Subsystem1/1(integSEB_input), If Action Subsystem2/1(integSEB_input), If Action Subsystem/1(integSEB_input)
  pitch_dem_1/1 -> If Action Subsystem1/3(pitch_dem)
  PITCHmaxf_1/1 -> If Action Subsystem/2(PITCHmaxf)
  If/3 -> If Action Subsystem2/Action
  PITCHmaxf/1 -> If/2
  Merge/1 -> y/1
  PITCHminf/1 -> If/3
  pitch_dem/1 -> If Action Subsystem/3(pitch_dem)
  If/1 -> If Action Subsystem/Action
  If/2 -> If Action Subsystem1/Action

== system Bixler/BIXLER DYNAMICS/RUBBISH BIN/TECS/PITCH1/integSEB ==
  temp : Inport
  gainInv : Inport  Port=2
  PITCHminf : Inport  Port=3
  PITCHmaxf : Inport  Port=4
  integSEB_delta : Inport  Port=5
  Constant : Constant  Value=0.0783
  Constant1 : Constant  Value=0.0783
  Gain : Gain  Gain=0.1
  Gain1 : Gain  Gain=-0.1
  Product : Product
  Product1 : Product
  Saturation Dynamic : simulink/Discontinuities/Saturation Dynamic  OutMin=[]  OutMax=[]  OutDataTypeStr=Inherit: Same as second input  OutDataType=fixdt(1, 16)  OutScaling=2^-10  DoSatur=off
  Sum{,1,3..4} (4 alike) : Sum  Inputs=|+-
  Sum2 : Sum  Inputs=|++
  gainInv_1 : InportShadow  Port=2
  temp_1 : InportShadow
  "IntegSEB_delta " : Outport  VectorParamsAs1DForOutWhenUnconnected=off
  "integSEB_min " : Outport  Port=2  VectorParamsAs1DForOutWhenUnconnected=off
  integSEB_max : Outport  Port=3  VectorParamsAs1DForOutWhenUnconnected=off
  wires:
  PITCHminf/1 -> Sum/1
  Product/1 -> Sum1/1
  Constant1/1 -> Sum2/2
  Sum3/1 -> integSEB_max/1, [integSEB_max]
  PITCHmaxf/1 -> Sum2/1
  Sum2/1 -> Product1/2
  Product1/1 -> Sum3/1
  gainInv_1/1 -> Product1/1
  temp_1/1 -> Sum3/2
  Constant/1 -> Sum/2
  integSEB_delta/1 -> Saturation Dynamic/2
  Sum/1 -> Product/2
  Sum1/1 -> "integSEB_min "/1, [integSEB_min]
  temp/1 -> Sum1/2
  [integSEB_range] -> Gain1/1
  Gain1/1 -> Saturation Dynamic/3
  Saturation Dynamic/1 -> "IntegSEB_delta "/1
  Sum4/1 -> [integSEB_range]
  [integSEB_min] -> Sum4/2
  [integSEB_max] -> Sum4/1
  [integSEB_range] -> Gain/1
  Gain/1 -> Saturation Dynamic/1
  gainInv/1 -> Product/1

== system Bixler/BIXLER DYNAMICS/RUBBISH BIN/TECS/PITCH1/timeConstant() ==
  Constant1 : Constant  Value=0.1
  Constant5 : Constant  Value=Ctr.TECS.TIME_CONST
  MinMax : MinMax  Function=max  Inputs=2
  timeConstant : Outport  VectorParamsAs1DForOutWhenUnconnected=off
  wires:
  MinMax/1 -> timeConstant/1
  Constant1/1 -> MinMax/2
  Constant5/1 -> MinMax/1

== system Bixler/BIXLER DYNAMICS/RUBBISH BIN/TECS/PITCH1/timeConstant()1 ==
  Constant1 : Constant  Value=0.1
  Constant5 : Constant  Value=Ctr.TECS.TIME_CONST
  MinMax : MinMax  Function=max  Inputs=2
  timeConstant : Outport  VectorParamsAs1DForOutWhenUnconnected=off
  wires:
  MinMax/1 -> timeConstant/1
  Constant1/1 -> MinMax/2
  Constant5/1 -> MinMax/1

== system Bixler/BIXLER DYNAMICS/Vehicle Airframe/Aerodynamics/Aerodynamic Coefficients/Forces ==
  note: CL
  note: Cy
  note: CD
  note: f_y is already in the body frame
  alpha_k : Inport
  alpha_f : Inport  Port=2
  CD interpolation : Interpolation_n-D  NumberOfTableDimensions=1  Table=Aero.CD_Basic  RemoveProtectionIndex=on  InternalRulePriority=Speed
      settings: InputPortMap=u0,u1
  CL interpolation : Interpolation_n-D  NumberOfTableDimensions=1  Table=Aero.CL_Basic  RemoveProtectionIndex=on  InternalRulePriority=Speed
      settings: InputPortMap=u0,u1
  CYp Interpolation : Interpolation_n-D  NumberOfTableDimensions=1  Table=Aero.Cy_RollRate  RemoveProtectionIndex=on  InternalRulePriority=Speed
      settings: InputPortMap=u0,u1
  Constant1 : Constant  Value=Aero.CL_PitchRate
  Constant6 : Constant  Value=Aero.Cy_Beta
  Divide1 : Product  Inputs=**/
  Divide3 : Product  Inputs=**
  Divide4 : Product  Inputs=**/
  Gain10 : Gain  Gain=2
  Gain2 : Gain  Gain=Bxl.c
  Gain3 : Gain  Gain=2
  Gain9 : Gain  Gain=Bxl.b
  Sum1 : Sum  Inputs=|++
  Sum3 : Sum  Inputs=++|
  CD : Outport  VectorParamsAs1DForOutWhenUnconnected=off
  Cy : Outport  Port=2  VectorParamsAs1DForOutWhenUnconnected=off
  CL : Outport  Port=3  VectorParamsAs1DForOutWhenUnconnected=off
  wires:
  Gain2/1 -> Divide1/1
  Constant1/1 -> Gain2/1
  Gain3/1 -> Divide1/3
  [Va] -> Gain3/1
  [qRad] -> Divide1/2  "q=pitch rate"
  Divide1/1 -> Sum1/2
  [pRad] -> Divide4/2  "q=roll rate"
  [Va] -> Gain10/1
  Gain9/1 -> Divide4/1
  Gain10/1 -> Divide4/3
  Sum3/1 -> Cy/1  "Cy"
  CL interpolation/1 -> Sum1/1  "CL(alpha)"
  CYp Interpolation/1 -> Gain9/1
  alpha_k/1 -> CL interpolation/1, CYp Interpolation/1, CD interpolation/1
  alpha_f/1 -> CL interpolation/2, CYp Interpolation/2, CD interpolation/2
  Divide4/1 -> Sum3/2
  CD interpolation/1 -> CD/1  "CD(alpha)"
  Sum1/1 -> CL/1  "CL"
  [BetaRad] -> Divide3/2
  Constant6/1 -> Divide3/1
  Divide3/1 -> Sum3/1
